simulink model "eVTOL_System"  (R2024b)
settings: Solver=FixedStepAuto  StartTime=0.0  StopTime=inf  RelTol=1e-3
undefined symbols (not defined in the file): airspeed, Battery, BCE12, BCE_Set_init, BMS_Controller_State, C, Cell10_P, Cell11_P, Cell12_P, Cell13_P, Cell14_P, Cell15_P, Cell16_P, Cell17_P, Cell18_P, Cell19_P, Cell1_N, Cell1_P, Cell20_P, Cell21_P, Cell22_P, Cell23_P, Cell24_P, Cell2_P, Cell3_P, Cell4_P, Cell5_P, Cell6_P, Cell7_P, Cell8_P, Cell9_P, Charging_State, CityMission, control, controlParams, ControlSampleTime, CriticalTiltAngle, currentFactor, CV_Gain, ddx, ddy, ddz, Device_01, Device_02, DiscIntNeverNeededParam, dx, dy, dz, Earth, env, F, F28379D_ADC_MaxCount, F28379D_ADC_Vmax, FixedWingMission, flightState, Foc_Ki_IxTcpu, Foc_Ki_S, Foc_Kp_I, Foc_Kp_S, fractalcoef ... (+68)
libraries: fl_lib x1115, nesl_utility x617, slrealtimeethercatlib x217, simulink x130, canmsglib x101, speedgoatlib_IO611_obsolete x91, slpidlib x49, mcbcontrolslib x44, slrealtimeutilitieslib x35, speedgoatlib_hdlCoder_IO3xx x31, dspstat3 x24, mcbpositiondecoderlib x12
(part 17 of 31)

== system eVTOL_System/Battery System/BMS/HIL/Controller_100Cells/PLANT-Rx/Messages ==
  ID_0x201 : Inport
  ID_0x202 : Inport  Port=2
  ID_0x501 : Inport  Port=3
  ID_0x502 : Inport  Port=4
  ID_0x203 : Inport  Port=5
  ID_0x204 : Inport  Port=6
  Balancing : simulink/Sources/Enumerated Constant  OutDataTypeStr=Enum: BMS_Controller_State  Value=BMS_Controller_State.BMS_Idle  SampleTime=-1
  Balancing1 : simulink/Sources/Enumerated Constant  OutDataTypeStr=Enum: Charging_State  Value=Charging_State.Init  SampleTime=-1
  Bus Creator : BusCreator  Inputs=5  OutDataTypeStr=Bus: Faults
  CAN Unpack : canmsglib/CAN Unpack  MsgList=(none)  MsgName=CAN Msg  MsgIDType=Standard (11-bit identifier)  MsgIdentifier=0x201  MsgLength=8  SignalInfo={ 'DischargeCurrentLimit_CAN', '0', '32', 'LE', 'single', 'Standard', '0', '1', '0', '-inf', '+inf'; 'ChargeCurrentLimit_CAN', '32', '32', 'LE', 'single', 'Standard', '0', '1', '0', '-Inf', 'Inf' }  IDPort=off  TimestampPort=on  ErrorPort=off  RemotePort=off  LengthPort=off  StatusPort=on  ApplyMinMax=off
      settings: LibrarySourceBlock=embeddedtargetslib/Host Communication/CAN Unpack
  CAN Unpack1 : canmsglib/CAN Unpack  MsgList=(none)  MsgName=CAN Msg  MsgIDType=Standard (11-bit identifier)  MsgIdentifier=0x202  MsgLength=4  SignalInfo={ 'ChargeCurrentReq', '0', '32', 'LE', 'single', 'Standard', '0', '1', '0', '-inf', '+inf' }  IDPort=off  TimestampPort=on  ErrorPort=off  RemotePort=off  LengthPort=off  StatusPort=on  ApplyMinMax=off
      settings: LibrarySourceBlock=embeddedtargetslib/Host Communication/CAN Unpack
  CAN Unpack2 : canmsglib/CAN Unpack  MsgList=(none)  MsgName=CAN Msg  MsgIDType=Standard (11-bit identifier)  MsgIdentifier=0x501  MsgLength=8  SignalInfo={ 'SOC_UKF', '0', '32', 'LE', 'single', 'Standard', '0', '1', '0', '-inf', '+inf'; 'SOC_EKF', '32', '32', 'LE', 'single', 'Standard', '0', '1', '0', '-Inf', 'Inf' }  IDPort=off  TimestampPort=on  ErrorPort=off  RemotePort=off  LengthPort=off  StatusPort=on  ApplyMinMax=off
      settings: LibrarySourceBlock=embeddedtargetslib/Host Communication/CAN Unpack
  CAN Unpack3 : canmsglib/CAN Unpack  MsgList=(none)  MsgName=CAN Msg  MsgIDType=Standard (11-bit identifier)  MsgIdentifier=0x502  MsgLength=7  SignalInfo={ 'SOC_CC', '0', '32', 'LE', 'single', 'Standard', '0', '1', '0', '-inf', '+inf'; 'Faults', '32', '8', 'LE', 'unsigned', 'Standard', '0', '1', '0', '-Inf', 'Inf'; 'BMS_State', '40', '8', 'LE', 'unsigned', 'Standard', '0', '1', '0', '-Inf', 'Inf'; 'Charging_State', '48', '8', 'LE', 'signed', 'Standard', '0', '1', '0', '-Inf', 'Inf' }  IDPort=off  TimestampPort=on  ErrorPort=off  RemotePort=off  LengthPort=off  StatusPort=on  ApplyMinMax=off
      settings: LibrarySourceBlock=embeddedtargetslib/Host Communication/CAN Unpack
  CAN Unpack4 : canmsglib/CAN Unpack  MsgList=(none)  MsgName=CAN Msg  MsgIDType=Standard (11-bit identifier)  MsgIdentifier=0x203  MsgLength=8  SignalInfo={ 'Bal_Cmd1', '0', '32', 'LE', 'single', 'Standard', '0', '1', '0', '-inf', '+inf'; 'Bal_Cmd2', '32', '32', 'LE', 'single', 'Standard', '0', '1', '0', '-Inf', 'Inf' }  IDPort=off  TimestampPort=on  ErrorPort=off  RemotePort=off  LengthPort=off  StatusPort=on  ApplyMinMax=off
      settings: LibrarySourceBlock=embeddedtargetslib/Host Communication/CAN Unpack
  CAN Unpack5 : canmsglib/CAN Unpack  MsgList=(none)  MsgName=CAN Msg  MsgIDType=Standard (11-bit identifier)  MsgIdentifier=0x204  MsgLength=4  SignalInfo={ 'Bal_Cmd3', '0', '32', 'LE', 'single', 'Standard', '0', '1', '0', '-inf', '+inf' }  IDPort=off  TimestampPort=on  ErrorPort=off  RemotePort=off  LengthPort=off  StatusPort=on  ApplyMinMax=off
      settings: LibrarySourceBlock=embeddedtargetslib/Host Communication/CAN Unpack
  Charging : simulink/Sources/Enumerated Constant  OutDataTypeStr=Enum: BMS_Controller_State  Value=BMS_Controller_State.BMS_Driving  SampleTime=-1
  Charging1 : simulink/Sources/Enumerated Constant  OutDataTypeStr=Enum: Charging_State  Value=Charging_State.CC  SampleTime=-1
  Driving : simulink/Sources/Enumerated Constant  OutDataTypeStr=Enum: BMS_Controller_State  Value=BMS_Controller_State.BMS_Charging  SampleTime=-1
  Driving1 : simulink/Sources/Enumerated Constant  OutDataTypeStr=Enum: BMS_Controller_State  Value=BMS_Controller_State.BMS_Fault  SampleTime=-1
  Driving2 : simulink/Sources/Enumerated Constant  OutDataTypeStr=Enum: Charging_State  Value=Charging_State.CV  SampleTime=-1
  Faults_unpacking : slrealtimeutilitieslib/Bit Unpacking  SignExtend=on  MaskBitPatterns={[7:7] [6:6] [5:5] [4:4] [3:3] [2:2] [1:1] [0:0]}  MaskPackDataType=uint8  MaskPackDataSize=[1]  MaskUnpackDataTypes={'boolean', 'boolean', 'boolean', 'boolean', 'boolean', 'boolean', 'boolean', 'boolean'}  MaskUnpackDataSizes={[1] [1] [1] [1] [1] [1] [1] [1]}
  Gain : Gain  Gain=100
  Gain1 : Gain  Gain=100
  Gain2 : Gain  Gain=100
  Multiport Switch1 : MultiPortSwitch  DataPortOrder=Zero-based contiguous  zeroidx=on  SaturateOnIntegerOverflow=off  InputSameDT=off
  Multiport Switch2 : MultiPortSwitch  DataPortOrder=Zero-based contiguous  Inputs=4  zeroidx=on  SaturateOnIntegerOverflow=off  InputSameDT=off
  Mux1 : Mux  Inputs=3
  Subsystem : Subsystem
  Terminator{,1..10,13..16} (15 alike) : Terminator
  Discharge_Current_Limit : Outport
  Charge_Current_Limit : Outport  Port=2
  Charge_Current_Req : Outport  Port=3
  SOC : Outport  Port=4
  BMS_Faults : Outport  Port=5
  BMS_State : Outport  Port=6
  Charging_State : Outport  Port=7
  Bal_Cmd_76Cells : Outport  Port=8
  wires:
  CAN Unpack1/2 -> Terminator2/1
  CAN Unpack/1 -> Discharge_Current_Limit/1  "Discharge_Current_Limit"
  CAN Unpack1/1 -> Charge_Current_Req/1  "Charge_Current_Req"
  CAN Unpack1/3 -> Terminator5/1
  CAN Unpack/2 -> Charge_Current_Limit/1  "Charge_Current_Limit"
  CAN Unpack/4 -> Terminator7/1
  CAN Unpack/3 -> Terminator4/1
  ID_0x201/1 -> CAN Unpack/1
  ID_0x202/1 -> CAN Unpack1/1
  CAN Unpack2/2 -> Gain1/1
  Bus Creator/1 -> BMS_Faults/1
  Faults_unpacking/5 -> Bus Creator/5  "UnderVolt"
  CAN Unpack3/5 -> Terminator10/1
  CAN Unpack3/3 -> Multiport Switch2/1
  CAN Unpack3/2 -> Faults_unpacking/1
  Faults_unpacking/4 -> Bus Creator/4  "OverVolt"
  Faults_unpacking/3 -> Bus Creator/3  "LowTemp"
  CAN Unpack2/1 -> Gain/1
  Faults_unpacking/1 -> Bus Creator/1  "OverCurrent"
  ID_0x501/1 -> CAN Unpack2/1
  Faults_unpacking/2 -> Bus Creator/2  "HighTemp"
  CAN Unpack2/3 -> Terminator/1  "Time_0x501"
  ID_0x502/1 -> CAN Unpack3/1
  Gain/1 -> Mux1/1  "SOC_UKF"
  Gain1/1 -> Mux1/2  "SOC_EKF"
  CAN Unpack3/1 -> Gain2/1
  CAN Unpack2/4 -> Terminator1/1  "Status_0x501"
  Faults_unpacking/6 -> Terminator13/1
  Faults_unpacking/7 -> Terminator14/1
  Faults_unpacking/8 -> Terminator15/1
  CAN Unpack3/6 -> Terminator16/1
  Gain2/1 -> Mux1/3  "SOC_CC"
  Mux1/1 -> SOC/1  "SOC"
  Charging/1 -> Multiport Switch2/3
  Balancing/1 -> Multiport Switch2/2
  Driving/1 -> Multiport Switch2/4
  Driving1/1 -> Multiport Switch2/5
  Charging1/1 -> Multiport Switch1/3
  Driving2/1 -> Multiport Switch1/4
  Balancing1/1 -> Multiport Switch1/2
  CAN Unpack3/4 -> Multiport Switch1/1
  Multiport Switch1/1 -> Charging_State/1
  Multiport Switch2/1 -> BMS_State/1
  ID_0x203/1 -> CAN Unpack4/1
  ID_0x204/1 -> CAN Unpack5/1
  CAN Unpack5/3 -> Terminator9/1
  CAN Unpack5/2 -> Terminator8/1
  CAN Unpack4/3 -> Terminator3/1
  CAN Unpack4/4 -> Terminator6/1
  CAN Unpack4/1 -> Subsystem/1(In1)
  CAN Unpack5/1 -> Subsystem/3(3)
  CAN Unpack4/2 -> Subsystem/2(In2)
  Subsystem/1(Bal_Cmd_76Cells) -> Bal_Cmd_76Cells/1

== system eVTOL_System/Battery System/BMS/HIL/Controller_100Cells/PLANT-Tx/24-Cell ==
  to_Controller : Inport
  to_Controller_SRE : Inport  Port=2
  100 cells Temperature : Subsystem
  76 cells Voltage : Subsystem
  Bus Selector : BusSelector  OutputSignals=Pack_Current,Cell_Temperatures,Pack_Voltage2
  CAN Pack4 : canmsglib/CAN Pack  MsgList=(none)  MsgName=CAN Msg  MsgIDType=Standard (11-bit identifier)  MsgIdentifier=0x401  CANIDInput=off  MsgLength=5  Remote=off  ApplyMinMax=off  BusOutput=off  SignalInfo={ 'Pack_Current', '0', '32', 'LE', 'single', 'Standard', '0', '1', '0', '-Inf', 'Inf'; 'SRE', '32', '8', 'LE', 'unsigned', 'Standard', '0', '1', '0', '-Inf', 'Inf' }
      settings: LibrarySourceBlock=embeddedtargetslib/Host Communication/CAN Pack  DataFormat=manually specified signals
  CAN Write : speedgoatlib_IO611_obsolete/CAN/CAN Write  id=1  sampleTime=-1  portSelection=2  messageType=CAN  BusInput=off  enaStatusPort=off  protl=IO611  ptIdx=1  isFDMod=1
      settings: SourceProductName=IO611
  Selector : Subsystem  Commented=on
  wires:
  to_Controller/1 -> Bus Selector/1
  Bus Selector/1 -> CAN Pack4/1  "<Pack_Current>"
  CAN Pack4/1 -> CAN Write/1
  to_Controller_SRE/1 -> CAN Pack4/2
  Bus Selector/2 -> 100 cells Temperature/1(In1)  "<Cell_Temperatures>"
  Bus Selector/3 -> 76 cells Voltage/1(In1)  "<Pack_Voltage2>"

== system eVTOL_System/Battery System/BMS/HIL/Controller_76Cells/BMS State Machine/Selector1 ==
  In1 : Inport
  Demux : Demux  Outputs=100
  Mux : Mux  Inputs=24
  Mux1 : Mux  Inputs=76
  Terminator : Terminator
  Out1 : Outport
  wires:
  In1/1 -> Demux/1
  Demux/1 -> Mux/1
  Demux/2 -> Mux/2
  Demux/3 -> Mux/3
  Demux/4 -> Mux/4
  Demux/5 -> Mux/5
  Demux/6 -> Mux/6
  Demux/7 -> Mux/7
  Demux/8 -> Mux/8
  Demux/9 -> Mux/9
  Demux/10 -> Mux/10
  Demux/11 -> Mux/11
  Demux/12 -> Mux/12
  Demux/13 -> Mux/13
  Demux/14 -> Mux/14
  Demux/15 -> Mux/15
  Demux/16 -> Mux/16
  Demux/17 -> Mux/17
  Demux/18 -> Mux/18
  Demux/19 -> Mux/19
  Demux/20 -> Mux/20
  Demux/21 -> Mux/21
  Demux/22 -> Mux/22
  Demux/23 -> Mux/23
  Demux/24 -> Mux/24
  Demux/25 -> Mux1/1
  Demux/26 -> Mux1/2
  Demux/27 -> Mux1/3
  Demux/28 -> Mux1/4
  Demux/29 -> Mux1/5
  Demux/30 -> Mux1/6
  Demux/31 -> Mux1/7
  Demux/32 -> Mux1/8
  Demux/33 -> Mux1/9
  Demux/34 -> Mux1/10
  Demux/35 -> Mux1/11
  Demux/36 -> Mux1/12
  Demux/37 -> Mux1/13
  Demux/38 -> Mux1/14
  Demux/39 -> Mux1/15
  Demux/40 -> Mux1/16
  Demux/41 -> Mux1/17
  Demux/42 -> Mux1/18
  Demux/43 -> Mux1/19
  Demux/44 -> Mux1/20
  Demux/45 -> Mux1/21
  Demux/46 -> Mux1/22
  Demux/47 -> Mux1/23
  Demux/48 -> Mux1/24
  Demux/49 -> Mux1/25
  Demux/50 -> Mux1/26
  Demux/51 -> Mux1/27
  Demux/52 -> Mux1/28
  Demux/53 -> Mux1/29
  Demux/54 -> Mux1/30
  Demux/55 -> Mux1/31
  Demux/56 -> Mux1/32
  Demux/57 -> Mux1/33
  Demux/58 -> Mux1/34
  Demux/59 -> Mux1/35
  Demux/60 -> Mux1/36
  Demux/61 -> Mux1/37
  Demux/62 -> Mux1/38
  Demux/63 -> Mux1/39
  Demux/64 -> Mux1/40
  Demux/65 -> Mux1/41
  Demux/66 -> Mux1/42
  Demux/67 -> Mux1/43
  Demux/68 -> Mux1/44
  Demux/69 -> Mux1/45
  Demux/70 -> Mux1/46
  Demux/71 -> Mux1/47
  Demux/72 -> Mux1/48
  Demux/73 -> Mux1/49
  Demux/74 -> Mux1/50
  Demux/75 -> Mux1/51
  Demux/76 -> Mux1/52
  Demux/77 -> Mux1/53
  Demux/78 -> Mux1/54
  Demux/79 -> Mux1/55
  Demux/80 -> Mux1/56
  Demux/81 -> Mux1/57
  Demux/82 -> Mux1/58
  Demux/83 -> Mux1/59
  Demux/84 -> Mux1/60
  Demux/85 -> Mux1/61
  Demux/86 -> Mux1/62
  Demux/87 -> Mux1/63
  Demux/88 -> Mux1/64
  Demux/89 -> Mux1/65
  Demux/90 -> Mux1/66
  Demux/91 -> Mux1/67
  Demux/92 -> Mux1/68
  Demux/93 -> Mux1/69
  Demux/94 -> Mux1/70
  Demux/95 -> Mux1/71
  Demux/96 -> Mux1/72
  Demux/97 -> Mux1/73
  Demux/98 -> Mux1/74
  Demux/99 -> Mux1/75
  Demux/100 -> Mux1/76
  Mux1/1 -> Out1/1
  Mux/1 -> Terminator/1

== system eVTOL_System/Battery System/BMS/HIL/Controller_76Cells/BMS State Machine/Selector3 ==
  In1 : Inport
  Demux : Demux  Outputs=100
  Mux : Mux  Inputs=24
  Mux1 : Mux  Inputs=76
  Terminator : Terminator
  Out1 : Outport
  wires:
  In1/1 -> Demux/1
  Demux/1 -> Mux/1
  Demux/2 -> Mux/2
  Demux/3 -> Mux/3
  Demux/4 -> Mux/4
  Demux/5 -> Mux/5
  Demux/6 -> Mux/6
  Demux/7 -> Mux/7
  Demux/8 -> Mux/8
  Demux/9 -> Mux/9
  Demux/10 -> Mux/10
  Demux/11 -> Mux/11
  Demux/12 -> Mux/12
  Demux/13 -> Mux/13
  Demux/14 -> Mux/14
  Demux/15 -> Mux/15
  Demux/16 -> Mux/16
  Demux/17 -> Mux/17
  Demux/18 -> Mux/18
  Demux/19 -> Mux/19
  Demux/20 -> Mux/20
  Demux/21 -> Mux/21
  Demux/22 -> Mux/22
  Demux/23 -> Mux/23
  Demux/24 -> Mux/24
  Demux/25 -> Mux1/1
  Demux/26 -> Mux1/2
  Demux/27 -> Mux1/3
  Demux/28 -> Mux1/4
  Demux/29 -> Mux1/5
  Demux/30 -> Mux1/6
  Demux/31 -> Mux1/7
  Demux/32 -> Mux1/8
  Demux/33 -> Mux1/9
  Demux/34 -> Mux1/10
  Demux/35 -> Mux1/11
  Demux/36 -> Mux1/12
  Demux/37 -> Mux1/13
  Demux/38 -> Mux1/14
  Demux/39 -> Mux1/15
  Demux/40 -> Mux1/16
  Demux/41 -> Mux1/17
  Demux/42 -> Mux1/18
  Demux/43 -> Mux1/19
  Demux/44 -> Mux1/20
  Demux/45 -> Mux1/21
  Demux/46 -> Mux1/22
  Demux/47 -> Mux1/23
  Demux/48 -> Mux1/24
  Demux/49 -> Mux1/25
  Demux/50 -> Mux1/26
  Demux/51 -> Mux1/27
  Demux/52 -> Mux1/28
  Demux/53 -> Mux1/29
  Demux/54 -> Mux1/30
  Demux/55 -> Mux1/31
  Demux/56 -> Mux1/32
  Demux/57 -> Mux1/33
  Demux/58 -> Mux1/34
  Demux/59 -> Mux1/35
  Demux/60 -> Mux1/36
  Demux/61 -> Mux1/37
  Demux/62 -> Mux1/38
  Demux/63 -> Mux1/39
  Demux/64 -> Mux1/40
  Demux/65 -> Mux1/41
  Demux/66 -> Mux1/42
  Demux/67 -> Mux1/43
  Demux/68 -> Mux1/44
  Demux/69 -> Mux1/45
  Demux/70 -> Mux1/46
  Demux/71 -> Mux1/47
  Demux/72 -> Mux1/48
  Demux/73 -> Mux1/49
  Demux/74 -> Mux1/50
  Demux/75 -> Mux1/51
  Demux/76 -> Mux1/52
  Demux/77 -> Mux1/53
  Demux/78 -> Mux1/54
  Demux/79 -> Mux1/55
  Demux/80 -> Mux1/56
  Demux/81 -> Mux1/57
  Demux/82 -> Mux1/58
  Demux/83 -> Mux1/59
  Demux/84 -> Mux1/60
  Demux/85 -> Mux1/61
  Demux/86 -> Mux1/62
  Demux/87 -> Mux1/63
  Demux/88 -> Mux1/64
  Demux/89 -> Mux1/65
  Demux/90 -> Mux1/66
  Demux/91 -> Mux1/67
  Demux/92 -> Mux1/68
  Demux/93 -> Mux1/69
  Demux/94 -> Mux1/70
  Demux/95 -> Mux1/71
  Demux/96 -> Mux1/72
  Demux/97 -> Mux1/73
  Demux/98 -> Mux1/74
  Demux/99 -> Mux1/75
  Demux/100 -> Mux1/76
  Mux1/1 -> Out1/1
  Mux/1 -> Terminator/1

== system eVTOL_System/Battery System/BMS/HIL/Controller_76Cells/Balancing Logic/Selector1 ==
  In1 : Inport
  Demux : Demux  Outputs=100
  Mux : Mux  Inputs=24
  Mux1 : Mux  Inputs=76
  Terminator : Terminator
  Out1 : Outport
  wires:
  In1/1 -> Demux/1
  Demux/1 -> Mux/1
  Demux/2 -> Mux/2
  Demux/3 -> Mux/3
  Demux/4 -> Mux/4
  Demux/5 -> Mux/5
  Demux/6 -> Mux/6
  Demux/7 -> Mux/7
  Demux/8 -> Mux/8
  Demux/9 -> Mux/9
  Demux/10 -> Mux/10
  Demux/11 -> Mux/11
  Demux/12 -> Mux/12
  Demux/13 -> Mux/13
  Demux/14 -> Mux/14
  Demux/15 -> Mux/15
  Demux/16 -> Mux/16
  Demux/17 -> Mux/17
  Demux/18 -> Mux/18
  Demux/19 -> Mux/19
  Demux/20 -> Mux/20
  Demux/21 -> Mux/21
  Demux/22 -> Mux/22
  Demux/23 -> Mux/23
  Demux/24 -> Mux/24
  Demux/25 -> Mux1/1
  Demux/26 -> Mux1/2
  Demux/27 -> Mux1/3
  Demux/28 -> Mux1/4
  Demux/29 -> Mux1/5
  Demux/30 -> Mux1/6
  Demux/31 -> Mux1/7
  Demux/32 -> Mux1/8
  Demux/33 -> Mux1/9
  Demux/34 -> Mux1/10
  Demux/35 -> Mux1/11
  Demux/36 -> Mux1/12
  Demux/37 -> Mux1/13
  Demux/38 -> Mux1/14
  Demux/39 -> Mux1/15
  Demux/40 -> Mux1/16
  Demux/41 -> Mux1/17
  Demux/42 -> Mux1/18
  Demux/43 -> Mux1/19
  Demux/44 -> Mux1/20
  Demux/45 -> Mux1/21
  Demux/46 -> Mux1/22
  Demux/47 -> Mux1/23
  Demux/48 -> Mux1/24
  Demux/49 -> Mux1/25
  Demux/50 -> Mux1/26
  Demux/51 -> Mux1/27
  Demux/52 -> Mux1/28
  Demux/53 -> Mux1/29
  Demux/54 -> Mux1/30
  Demux/55 -> Mux1/31
  Demux/56 -> Mux1/32
  Demux/57 -> Mux1/33
  Demux/58 -> Mux1/34
  Demux/59 -> Mux1/35
  Demux/60 -> Mux1/36
  Demux/61 -> Mux1/37
  Demux/62 -> Mux1/38
  Demux/63 -> Mux1/39
  Demux/64 -> Mux1/40
  Demux/65 -> Mux1/41
  Demux/66 -> Mux1/42
  Demux/67 -> Mux1/43
  Demux/68 -> Mux1/44
  Demux/69 -> Mux1/45
  Demux/70 -> Mux1/46
  Demux/71 -> Mux1/47
  Demux/72 -> Mux1/48
  Demux/73 -> Mux1/49
  Demux/74 -> Mux1/50
  Demux/75 -> Mux1/51
  Demux/76 -> Mux1/52
  Demux/77 -> Mux1/53
  Demux/78 -> Mux1/54
  Demux/79 -> Mux1/55
  Demux/80 -> Mux1/56
  Demux/81 -> Mux1/57
  Demux/82 -> Mux1/58
  Demux/83 -> Mux1/59
  Demux/84 -> Mux1/60
  Demux/85 -> Mux1/61
  Demux/86 -> Mux1/62
  Demux/87 -> Mux1/63
  Demux/88 -> Mux1/64
  Demux/89 -> Mux1/65
  Demux/90 -> Mux1/66
  Demux/91 -> Mux1/67
  Demux/92 -> Mux1/68
  Demux/93 -> Mux1/69
  Demux/94 -> Mux1/70
  Demux/95 -> Mux1/71
  Demux/96 -> Mux1/72
  Demux/97 -> Mux1/73
  Demux/98 -> Mux1/74
  Demux/99 -> Mux1/75
  Demux/100 -> Mux1/76
  Mux1/1 -> Out1/1
  Mux/1 -> Terminator/1

== system eVTOL_System/Battery System/BMS/HIL/Controller_76Cells/Current Calculations/Charge_Current_Limit_Calc ==
  MaxCellVolt : Inport
  MinCellTemp : Inport  Port=2
  MaxCellTemp : Inport  Port=3
  Divide1 : Product  Inputs=*/
  HighTempChrgCurrentLim : Lookup_n-D  NumberOfTableDimensions=1  BreakpointsForDimension1=273.15+[-30:1:70]  Table=50*(1-tanh(273.15+[-30:1:70]-273.15-50))/2  InternalRulePriority=Speed  RndMeth=Simplest
  InternalCellResistance : Constant  Value=single(max(max(Battery(1).R0_LUT)))  OutDataTypeStr=single  SampleTime=-1
  LowTempChrgCurrentLim : Lookup_n-D  NumberOfTableDimensions=1  BreakpointsForDimension1=273.15+[-30:1:70]  Table=50*(1+tanh(273.15+[-30:1:70]-(273.15)))/2  InternalRulePriority=Speed  RndMeth=Simplest
  MinMax2 : MinMax  Inputs=3
  OverVoltageLimit : Constant  Value=OverCellVoltageLimit  OutDataTypeStr=single  SampleTime=-1
  Subtract1 : Sum  Inputs=+-
  Charge_Current_Limit : Outport  VectorParamsAs1DForOutWhenUnconnected=off
  wires:
  OverVoltageLimit/1 -> Subtract1/1
  MinMax2/1 -> Charge_Current_Limit/1  "ChargeCurrentLimit"
  MaxCellVolt/1 -> Subtract1/2
  Subtract1/1 -> Divide1/1
  Divide1/1 -> MinMax2/1
  InternalCellResistance/1 -> Divide1/2
  MinCellTemp/1 -> LowTempChrgCurrentLim/1
  MaxCellTemp/1 -> HighTempChrgCurrentLim/1
  HighTempChrgCurrentLim/1 -> MinMax2/3
  LowTempChrgCurrentLim/1 -> MinMax2/2

== system eVTOL_System/Battery System/BMS/HIL/Controller_76Cells/Current Calculations/Discharge_Current_Limit_Calc ==
  MinCellVolt : Inport
  MinCellTemp : Inport  Port=2
  MaxCellTemp : Inport  Port=3
  Divide : Product  Inputs=*/
  Gain : Gain  Gain=-1
  HighTempDchrgCurrentLim : Lookup_n-D  NumberOfTableDimensions=1  BreakpointsForDimension1=273.15+[-30:1:70]  Table=100*(1-tanh(273.15+[-30:1:70]-273.15-50))/2  InternalRulePriority=Speed  RndMeth=Simplest
  InternalCellResistance : Constant  Value=single(max(max(Battery(1).R0_LUT)))  OutDataTypeStr=single  SampleTime=-1
  LowTempDchrgCurrentLim : Lookup_n-D  NumberOfTableDimensions=1  BreakpointsForDimension1=273.15+[-30:1:70]  Table=100*(1+tanh(273.15+[-30:1:70]-(273.15)))/2  InternalRulePriority=Speed  RndMeth=Simplest
  MinMax2 : MinMax  Inputs=3
  Subtract : Sum  Inputs=+-
  UnderVoltageLimit : Constant  Value=UnderCellVoltageLimit  OutDataTypeStr=single  SampleTime=-1
  Discharge_Current_Limit : Outport  VectorParamsAs1DForOutWhenUnconnected=off
  wires:
  MinMax2/1 -> Gain/1  "DischargeCurrentLimit"
  Divide/1 -> MinMax2/1
  MinCellVolt/1 -> Subtract/1
  InternalCellResistance/1 -> Divide/2
  Subtract/1 -> Divide/1
  UnderVoltageLimit/1 -> Subtract/2
  Gain/1 -> Discharge_Current_Limit/1
  MaxCellTemp/1 -> HighTempDchrgCurrentLim/1
  MinCellTemp/1 -> LowTempDchrgCurrentLim/1
  HighTempDchrgCurrentLim/1 -> MinMax2/3
  LowTempDchrgCurrentLim/1 -> MinMax2/2

== system eVTOL_System/Battery System/BMS/HIL/Controller_76Cells/Current Calculations/Selector1 ==
  In1 : Inport
  Demux : Demux  Outputs=100
  Mux : Mux  Inputs=24
  Mux1 : Mux  Inputs=76
  Terminator : Terminator
  Out1 : Outport
  wires:
  In1/1 -> Demux/1
  Demux/1 -> Mux/1
  Demux/2 -> Mux/2
  Demux/3 -> Mux/3
  Demux/4 -> Mux/4
  Demux/5 -> Mux/5
  Demux/6 -> Mux/6
  Demux/7 -> Mux/7
  Demux/8 -> Mux/8
  Demux/9 -> Mux/9
  Demux/10 -> Mux/10
  Demux/11 -> Mux/11
  Demux/12 -> Mux/12
  Demux/13 -> Mux/13
  Demux/14 -> Mux/14
  Demux/15 -> Mux/15
  Demux/16 -> Mux/16
  Demux/17 -> Mux/17
  Demux/18 -> Mux/18
  Demux/19 -> Mux/19
  Demux/20 -> Mux/20
  Demux/21 -> Mux/21
  Demux/22 -> Mux/22
  Demux/23 -> Mux/23
  Demux/24 -> Mux/24
  Demux/25 -> Mux1/1
  Demux/26 -> Mux1/2
  Demux/27 -> Mux1/3
  Demux/28 -> Mux1/4
  Demux/29 -> Mux1/5
  Demux/30 -> Mux1/6
  Demux/31 -> Mux1/7
  Demux/32 -> Mux1/8
  Demux/33 -> Mux1/9
  Demux/34 -> Mux1/10
  Demux/35 -> Mux1/11
  Demux/36 -> Mux1/12
  Demux/37 -> Mux1/13
  Demux/38 -> Mux1/14
  Demux/39 -> Mux1/15
  Demux/40 -> Mux1/16
  Demux/41 -> Mux1/17
  Demux/42 -> Mux1/18
  Demux/43 -> Mux1/19
  Demux/44 -> Mux1/20
  Demux/45 -> Mux1/21
  Demux/46 -> Mux1/22
  Demux/47 -> Mux1/23
  Demux/48 -> Mux1/24
  Demux/49 -> Mux1/25
  Demux/50 -> Mux1/26
  Demux/51 -> Mux1/27
  Demux/52 -> Mux1/28
  Demux/53 -> Mux1/29
  Demux/54 -> Mux1/30
  Demux/55 -> Mux1/31
  Demux/56 -> Mux1/32
  Demux/57 -> Mux1/33
  Demux/58 -> Mux1/34
  Demux/59 -> Mux1/35
  Demux/60 -> Mux1/36
  Demux/61 -> Mux1/37
  Demux/62 -> Mux1/38
  Demux/63 -> Mux1/39
  Demux/64 -> Mux1/40
  Demux/65 -> Mux1/41
  Demux/66 -> Mux1/42
  Demux/67 -> Mux1/43
  Demux/68 -> Mux1/44
  Demux/69 -> Mux1/45
  Demux/70 -> Mux1/46
  Demux/71 -> Mux1/47
  Demux/72 -> Mux1/48
  Demux/73 -> Mux1/49
  Demux/74 -> Mux1/50
  Demux/75 -> Mux1/51
  Demux/76 -> Mux1/52
  Demux/77 -> Mux1/53
  Demux/78 -> Mux1/54
  Demux/79 -> Mux1/55
  Demux/80 -> Mux1/56
  Demux/81 -> Mux1/57
  Demux/82 -> Mux1/58
  Demux/83 -> Mux1/59
  Demux/84 -> Mux1/60
  Demux/85 -> Mux1/61
  Demux/86 -> Mux1/62
  Demux/87 -> Mux1/63
  Demux/88 -> Mux1/64
  Demux/89 -> Mux1/65
  Demux/90 -> Mux1/66
  Demux/91 -> Mux1/67
  Demux/92 -> Mux1/68
  Demux/93 -> Mux1/69
  Demux/94 -> Mux1/70
  Demux/95 -> Mux1/71
  Demux/96 -> Mux1/72
  Demux/97 -> Mux1/73
  Demux/98 -> Mux1/74
  Demux/99 -> Mux1/75
  Demux/100 -> Mux1/76
  Mux1/1 -> Out1/1
  Mux/1 -> Terminator/1

== system eVTOL_System/Battery System/BMS/HIL/Controller_76Cells/Current Calculations/Selector3 ==
  In1 : Inport
  Demux : Demux  Outputs=100
  Mux : Mux  Inputs=24
  Mux1 : Mux  Inputs=76
  Terminator : Terminator
  Out1 : Outport
  wires:
  In1/1 -> Demux/1
  Demux/1 -> Mux/1
  Demux/2 -> Mux/2
  Demux/3 -> Mux/3
  Demux/4 -> Mux/4
  Demux/5 -> Mux/5
  Demux/6 -> Mux/6
  Demux/7 -> Mux/7
  Demux/8 -> Mux/8
  Demux/9 -> Mux/9
  Demux/10 -> Mux/10
  Demux/11 -> Mux/11
  Demux/12 -> Mux/12
  Demux/13 -> Mux/13
  Demux/14 -> Mux/14
  Demux/15 -> Mux/15
  Demux/16 -> Mux/16
  Demux/17 -> Mux/17
  Demux/18 -> Mux/18
  Demux/19 -> Mux/19
  Demux/20 -> Mux/20
  Demux/21 -> Mux/21
  Demux/22 -> Mux/22
  Demux/23 -> Mux/23
  Demux/24 -> Mux/24
  Demux/25 -> Mux1/1
  Demux/26 -> Mux1/2
  Demux/27 -> Mux1/3
  Demux/28 -> Mux1/4
  Demux/29 -> Mux1/5
  Demux/30 -> Mux1/6
  Demux/31 -> Mux1/7
  Demux/32 -> Mux1/8
  Demux/33 -> Mux1/9
  Demux/34 -> Mux1/10
  Demux/35 -> Mux1/11
  Demux/36 -> Mux1/12
  Demux/37 -> Mux1/13
  Demux/38 -> Mux1/14
  Demux/39 -> Mux1/15
  Demux/40 -> Mux1/16
  Demux/41 -> Mux1/17
  Demux/42 -> Mux1/18
  Demux/43 -> Mux1/19
  Demux/44 -> Mux1/20
  Demux/45 -> Mux1/21
  Demux/46 -> Mux1/22
  Demux/47 -> Mux1/23
  Demux/48 -> Mux1/24
  Demux/49 -> Mux1/25
  Demux/50 -> Mux1/26
  Demux/51 -> Mux1/27
  Demux/52 -> Mux1/28
  Demux/53 -> Mux1/29
  Demux/54 -> Mux1/30
  Demux/55 -> Mux1/31
  Demux/56 -> Mux1/32
  Demux/57 -> Mux1/33
  Demux/58 -> Mux1/34
  Demux/59 -> Mux1/35
  Demux/60 -> Mux1/36
  Demux/61 -> Mux1/37
  Demux/62 -> Mux1/38
  Demux/63 -> Mux1/39
  Demux/64 -> Mux1/40
  Demux/65 -> Mux1/41
  Demux/66 -> Mux1/42
  Demux/67 -> Mux1/43
  Demux/68 -> Mux1/44
  Demux/69 -> Mux1/45
  Demux/70 -> Mux1/46
  Demux/71 -> Mux1/47
  Demux/72 -> Mux1/48
  Demux/73 -> Mux1/49
  Demux/74 -> Mux1/50
  Demux/75 -> Mux1/51
  Demux/76 -> Mux1/52
  Demux/77 -> Mux1/53
  Demux/78 -> Mux1/54
  Demux/79 -> Mux1/55
  Demux/80 -> Mux1/56
  Demux/81 -> Mux1/57
  Demux/82 -> Mux1/58
  Demux/83 -> Mux1/59
  Demux/84 -> Mux1/60
  Demux/85 -> Mux1/61
  Demux/86 -> Mux1/62
  Demux/87 -> Mux1/63
  Demux/88 -> Mux1/64
  Demux/89 -> Mux1/65
  Demux/90 -> Mux1/66
  Demux/91 -> Mux1/67
  Demux/92 -> Mux1/68
  Demux/93 -> Mux1/69
  Demux/94 -> Mux1/70
  Demux/95 -> Mux1/71
  Demux/96 -> Mux1/72
  Demux/97 -> Mux1/73
  Demux/98 -> Mux1/74
  Demux/99 -> Mux1/75
  Demux/100 -> Mux1/76
  Mux1/1 -> Out1/1
  Mux/1 -> Terminator/1

== system eVTOL_System/Battery System/BMS/HIL/Controller_76Cells/SOC Calculation/Coulomb Counting ==
  Curr : Inport
  Temp : Inport  Port=2
  1-D Lookup Table : Lookup_n-D  NumberOfTableDimensions=1  BreakpointsForDimension1=single(Battery(1).Temperature_LUT)  Table=single(Battery(1).Capacity_LUT)  InternalRulePriority=Speed  RndMeth=Simplest
  Discrete-Time Integrator : DiscreteIntegrator  InitialCondition=single(SOCInit+0.05)  SampleTime=-1  LimitOutput=on  UpperSaturationLimit=1  LowerSaturationLimit=0  ICPrevOutput=DiscIntNeverNeededParam  ICPrevScaledInput=DiscIntNeverNeededParam
  Divide : Product  Inputs=*/
  Gain : Gain  Gain=single(1/3600)
  SOC : Outport  VectorParamsAs1DForOutWhenUnconnected=off
  wires:
  Discrete-Time Integrator/1 -> SOC/1
  Curr/1 -> Gain/1
  Gain/1 -> Divide/1
  Divide/1 -> Discrete-Time Integrator/1
  1-D Lookup Table/1 -> Divide/2  "Capacity"
  Temp/1 -> 1-D Lookup Table/1

== system eVTOL_System/Battery System/BMS/HIL/Controller_76Cells/SOC Calculation/Measurement Function ==
  Current : Inport
  Temperature (K) : Inport  Port=2
  batteryMeasurementFcn : TriggerPort  TriggerType=function-call  IsSimulinkFunction=on  FunctionName=batteryMeasurementFcn  VariantControl=Variant
  Add1 : Sum  Inputs=+--
  Em Table : Lookup_n-D  BreakpointsForDimension1=Battery.SOC_LUT  BreakpointsForDimension2=Battery.Temperature_LUT  BeginIndexSearchUsingPreviousIndexResult=on  Table=Battery.Em_LUT  ExtrapMethod=Clip  InternalRulePriority=Speed  RndMeth=Simplest
      settings: InputPortMap=u0,u1
  Get SOC : Selector  InputPortWidth=2  IndexOptions=Index vector (dialog)  Indices=[1]  OutputSizes=1
  Get U1 : Selector  InputPortWidth=2  IndexOptions=Index vector (dialog)  Indices=2  OutputSizes=1
  Product : Product
  R0 Table : Lookup_n-D  BreakpointsForDimension1=Battery.SOC_LUT  BreakpointsForDimension2=Battery.Temperature_LUT  BeginIndexSearchUsingPreviousIndexResult=on  Table=Battery.R0_LUT  ExtrapMethod=Clip  InternalRulePriority=Speed  RndMeth=Simplest
      settings: InputPortMap=u0,u1
  x : ArgIn  DisableCoverage=on  OutDataTypeStr=single  PortDimensions=2  ArgumentName=x
  y : ArgOut  DisableCoverage=on  OutDataTypeStr=single  ArgumentName=y
  wires:
  Get U1/1 -> Add1/3  "U1"
  Product/1 -> Add1/2
  Current/1 -> Product/2
  R0 Table/1 -> Product/1
  Temperature (K)/1 -> Em Table/2, R0 Table/2
  Add1/1 -> y/1
  Em Table/1 -> Add1/1
  Get SOC/1 -> Em Table/1, R0 Table/1  "SOC"
  x/1 -> Get SOC/1, Get U1/1

== system eVTOL_System/Battery System/BMS/HIL/Controller_76Cells/SOC Calculation/Selector ==
  In1 : Inport
  Demux : Demux  Outputs=100
  Mux : Mux  Inputs=24
  Mux1 : Mux  Inputs=76
  Terminator : Terminator
  Out1 : Outport
  wires:
  In1/1 -> Demux/1
  Demux/1 -> Mux/1
  Demux/2 -> Mux/2
  Demux/3 -> Mux/3
  Demux/4 -> Mux/4
  Demux/5 -> Mux/5
  Demux/6 -> Mux/6
  Demux/7 -> Mux/7
  Demux/8 -> Mux/8
  Demux/9 -> Mux/9
  Demux/10 -> Mux/10
  Demux/11 -> Mux/11
  Demux/12 -> Mux/12
  Demux/13 -> Mux/13
  Demux/14 -> Mux/14
  Demux/15 -> Mux/15
  Demux/16 -> Mux/16
  Demux/17 -> Mux/17
  Demux/18 -> Mux/18
  Demux/19 -> Mux/19
  Demux/20 -> Mux/20
  Demux/21 -> Mux/21
  Demux/22 -> Mux/22
  Demux/23 -> Mux/23
  Demux/24 -> Mux/24
  Demux/25 -> Mux1/1
  Demux/26 -> Mux1/2
  Demux/27 -> Mux1/3
  Demux/28 -> Mux1/4
  Demux/29 -> Mux1/5
  Demux/30 -> Mux1/6
  Demux/31 -> Mux1/7
  Demux/32 -> Mux1/8
  Demux/33 -> Mux1/9
  Demux/34 -> Mux1/10
  Demux/35 -> Mux1/11
  Demux/36 -> Mux1/12
  Demux/37 -> Mux1/13
  Demux/38 -> Mux1/14
  Demux/39 -> Mux1/15
  Demux/40 -> Mux1/16
  Demux/41 -> Mux1/17
  Demux/42 -> Mux1/18
  Demux/43 -> Mux1/19
  Demux/44 -> Mux1/20
  Demux/45 -> Mux1/21
  Demux/46 -> Mux1/22
  Demux/47 -> Mux1/23
  Demux/48 -> Mux1/24
  Demux/49 -> Mux1/25
  Demux/50 -> Mux1/26
  Demux/51 -> Mux1/27
  Demux/52 -> Mux1/28
  Demux/53 -> Mux1/29
  Demux/54 -> Mux1/30
  Demux/55 -> Mux1/31
  Demux/56 -> Mux1/32
  Demux/57 -> Mux1/33
  Demux/58 -> Mux1/34
  Demux/59 -> Mux1/35
  Demux/60 -> Mux1/36
  Demux/61 -> Mux1/37
  Demux/62 -> Mux1/38
  Demux/63 -> Mux1/39
  Demux/64 -> Mux1/40
  Demux/65 -> Mux1/41
  Demux/66 -> Mux1/42
  Demux/67 -> Mux1/43
  Demux/68 -> Mux1/44
  Demux/69 -> Mux1/45
  Demux/70 -> Mux1/46
  Demux/71 -> Mux1/47
  Demux/72 -> Mux1/48
  Demux/73 -> Mux1/49
  Demux/74 -> Mux1/50
  Demux/75 -> Mux1/51
  Demux/76 -> Mux1/52
  Demux/77 -> Mux1/53
  Demux/78 -> Mux1/54
  Demux/79 -> Mux1/55
  Demux/80 -> Mux1/56
  Demux/81 -> Mux1/57
  Demux/82 -> Mux1/58
  Demux/83 -> Mux1/59
  Demux/84 -> Mux1/60
  Demux/85 -> Mux1/61
  Demux/86 -> Mux1/62
  Demux/87 -> Mux1/63
  Demux/88 -> Mux1/64
  Demux/89 -> Mux1/65
  Demux/90 -> Mux1/66
  Demux/91 -> Mux1/67
  Demux/92 -> Mux1/68
  Demux/93 -> Mux1/69
  Demux/94 -> Mux1/70
  Demux/95 -> Mux1/71
  Demux/96 -> Mux1/72
  Demux/97 -> Mux1/73
  Demux/98 -> Mux1/74
  Demux/99 -> Mux1/75
  Demux/100 -> Mux1/76
  Mux1/1 -> Out1/1
  Mux/1 -> Terminator/1

== system eVTOL_System/Battery System/BMS/HIL/Controller_76Cells/SOC Calculation/Selector1 ==
  In1 : Inport
  Demux : Demux  Outputs=100
  Mux : Mux  Inputs=24
  Mux1 : Mux  Inputs=76
  Terminator : Terminator
  Out1 : Outport
  wires:
  In1/1 -> Demux/1
  Demux/1 -> Mux/1
  Demux/2 -> Mux/2
  Demux/3 -> Mux/3
  Demux/4 -> Mux/4
  Demux/5 -> Mux/5
  Demux/6 -> Mux/6
  Demux/7 -> Mux/7
  Demux/8 -> Mux/8
  Demux/9 -> Mux/9
  Demux/10 -> Mux/10
  Demux/11 -> Mux/11
  Demux/12 -> Mux/12
  Demux/13 -> Mux/13
  Demux/14 -> Mux/14
  Demux/15 -> Mux/15
  Demux/16 -> Mux/16
  Demux/17 -> Mux/17
  Demux/18 -> Mux/18
  Demux/19 -> Mux/19
  Demux/20 -> Mux/20
  Demux/21 -> Mux/21
  Demux/22 -> Mux/22
  Demux/23 -> Mux/23
  Demux/24 -> Mux/24
  Demux/25 -> Mux1/1
  Demux/26 -> Mux1/2
  Demux/27 -> Mux1/3
  Demux/28 -> Mux1/4
  Demux/29 -> Mux1/5
  Demux/30 -> Mux1/6
  Demux/31 -> Mux1/7
  Demux/32 -> Mux1/8
  Demux/33 -> Mux1/9
  Demux/34 -> Mux1/10
  Demux/35 -> Mux1/11
  Demux/36 -> Mux1/12
  Demux/37 -> Mux1/13
  Demux/38 -> Mux1/14
  Demux/39 -> Mux1/15
  Demux/40 -> Mux1/16
  Demux/41 -> Mux1/17
  Demux/42 -> Mux1/18
  Demux/43 -> Mux1/19
  Demux/44 -> Mux1/20
  Demux/45 -> Mux1/21
  Demux/46 -> Mux1/22
  Demux/47 -> Mux1/23
  Demux/48 -> Mux1/24
  Demux/49 -> Mux1/25
  Demux/50 -> Mux1/26
  Demux/51 -> Mux1/27
  Demux/52 -> Mux1/28
  Demux/53 -> Mux1/29
  Demux/54 -> Mux1/30
  Demux/55 -> Mux1/31
  Demux/56 -> Mux1/32
  Demux/57 -> Mux1/33
  Demux/58 -> Mux1/34
  Demux/59 -> Mux1/35
  Demux/60 -> Mux1/36
  Demux/61 -> Mux1/37
  Demux/62 -> Mux1/38
  Demux/63 -> Mux1/39
  Demux/64 -> Mux1/40
  Demux/65 -> Mux1/41
  Demux/66 -> Mux1/42
  Demux/67 -> Mux1/43
  Demux/68 -> Mux1/44
  Demux/69 -> Mux1/45
  Demux/70 -> Mux1/46
  Demux/71 -> Mux1/47
  Demux/72 -> Mux1/48
  Demux/73 -> Mux1/49
  Demux/74 -> Mux1/50
  Demux/75 -> Mux1/51
  Demux/76 -> Mux1/52
  Demux/77 -> Mux1/53
  Demux/78 -> Mux1/54
  Demux/79 -> Mux1/55
  Demux/80 -> Mux1/56
  Demux/81 -> Mux1/57
  Demux/82 -> Mux1/58
  Demux/83 -> Mux1/59
  Demux/84 -> Mux1/60
  Demux/85 -> Mux1/61
  Demux/86 -> Mux1/62
  Demux/87 -> Mux1/63
  Demux/88 -> Mux1/64
  Demux/89 -> Mux1/65
  Demux/90 -> Mux1/66
  Demux/91 -> Mux1/67
  Demux/92 -> Mux1/68
  Demux/93 -> Mux1/69
  Demux/94 -> Mux1/70
  Demux/95 -> Mux1/71
  Demux/96 -> Mux1/72
  Demux/97 -> Mux1/73
  Demux/98 -> Mux1/74
  Demux/99 -> Mux1/75
  Demux/100 -> Mux1/76
  Mux1/1 -> Out1/1
  Mux/1 -> Terminator/1

== system eVTOL_System/Battery System/BMS/HIL/Controller_76Cells/SOC Calculation/State Transition Function ==
  Current : Inport
  Temperature K : Inport  Port=2
  batteryStateFcn : TriggerPort  TriggerType=function-call  IsSimulinkFunction=on  FunctionName=batteryStateFcn  VariantControl=Variant
  Add : Sum
  Add1 : Sum  Inputs=-+
  C1 : Lookup_n-D  BreakpointsForDimension1=Battery.SOC_LUT  BreakpointsForDimension2=Battery.Temperature_LUT  BeginIndexSearchUsingPreviousIndexResult=on  Table=Battery.C1_LUT  ExtrapMethod=Clip  InternalRulePriority=Speed  RndMeth=Simplest
      settings: InputPortMap=u0,u1
  Constant : Constant  Value=single(ts_system)  OutDataTypeStr=single
  Divide : Product  Inputs=*/
  Divide1 : Product  Inputs=*/
  Divide2 : Product  Inputs=*/
  Gain : Gain  Gain=-3600
  Get SOC : Selector  InputPortWidth=2  IndexOptions=Index vector (dialog)  Indices=1  OutputSizes=1
  Get U1 : Selector  InputPortWidth=2  IndexOptions=Index vector (dialog)  Indices=2  OutputSizes=1
  Lookup Table : Lookup_n-D  NumberOfTableDimensions=1  BreakpointsForDimension1=Battery.Temperature_LUT  BeginIndexSearchUsingPreviousIndexResult=on  Table=Battery.Capacity_LUT  InternalRulePriority=Speed  RndMeth=Simplest
  Mux : Mux  Inputs=2
  Product : Product  OutDataTypeStr=single
  Product1 : Product
  R1 : Lookup_n-D  BreakpointsForDimension1=Battery.SOC_LUT  BreakpointsForDimension2=Battery.Temperature_LUT  BeginIndexSearchUsingPreviousIndexResult=on  Table=Battery.R1_LUT  ExtrapMethod=Clip  InternalRulePriority=Speed  RndMeth=Simplest
      settings: InputPortMap=u0,u1
  x : ArgIn  DisableCoverage=on  OutDataTypeStr=single  PortDimensions=2  ArgumentName=x
  xNext : ArgOut  DisableCoverage=on  OutDataTypeStr=single  PortDimensions=2  ArgumentName=xNext
  wires:
  Lookup Table/1 -> Gain/1  "Cq"
  Product/1 -> Add/2
  Constant/1 -> Product/2
  Current/1 -> Divide1/1, Divide/1  "Current"
  Get SOC/1 -> C1/1, R1/1
  Temperature K/1 -> Lookup Table/1, C1/2, R1/2
  Add/1 -> xNext/1
  x/1 -> Add/1, Get U1/1, Get SOC/1
  Gain/1 -> Divide/2
  Divide/1 -> Mux/1  "xdot_1"
  Get U1/1 -> Divide2/1  "U1"
  Product1/1 -> Divide2/2  "R1*C1"
  R1/1 -> Product1/1  "R1"
  C1/1 -> Product1/2, Divide1/2  "C1"
  Divide1/1 -> Add1/2  "Current/C1"
  Divide2/1 -> Add1/1
  Add1/1 -> Mux/2  "xdot_2"
  Mux/1 -> Product/1  "xdot"

== system eVTOL_System/Battery System/BMS/HIL/Controller_76Cells/SOC Calculation/UKF_EKF_1TC ==
  Cell_Voltage : Inport
  Enable : EnablePort
  EKF : sharedTrackingLibrary/Extended Kalman Filter  StateTransitionFcn=batteryStateFcn  HasStateTransitionJacobianFcn=off  HasAdditiveProcessNoise=Additive  ProcessNoise=1e-10*eye(2)  HasTimeVaryingProcessNoise=off  HasStateTransitionFcnExtraArgument=0  InitialState=[single(SOCInit+0.05); 0;]  InitialStateCovariance=[1e-5 1]  MeasurementFcn1=batteryMeasurementFcn  HasMeasurementJacobianFcn1=off  HasMeasurementEnablePort1=off  HasAdditiveMeasurementNoise1=Additive  MeasurementNoise1=1e-1  HasTimeVaryingMeasurementNoise1=off  HasMeasurementFcnExtraArgument1=0  HasMeasurementWrapping1=off  MeasurementFcn2=myMeasurementFcn  HasMeasurementJacobianFcn2=off  HasMeasurementEnablePort2=off  HasAdditiveMeasurementNoise2=Additive  MeasurementNoise2=1  HasTimeVaryingMeasurementNoise2=off  HasMeasurementFcnExtraArgument2=0  HasMeasurementWrapping2=off  MeasurementFcn3=myMeasurementFcn  HasMeasurementJacobianFcn3=off  HasMeasurementEnablePort3=off  HasAdditiveMeasurementNoise3=Additive  MeasurementNoise3=1  HasTimeVaryingMeasurementNoise3=off  HasMeasurementFcnExtraArgument3=0  HasMeasurementWrapping3=off  MeasurementFcn4=myMeasurementFcn  HasMeasurementJacobianFcn4=off  HasMeasurementEnablePort4=off  HasAdditiveMeasurementNoise4=Additive  MeasurementNoise4=1  HasTimeVaryingMeasurementNoise4=off  HasMeasurementFcnExtraArgument4=0  HasMeasurementWrapping4=off  MeasurementFcn5=myMeasurementFcn  HasMeasurementJacobianFcn5=off  HasMeasurementEnablePort5=off  HasAdditiveMeasurementNoise5=Additive  MeasurementNoise5=1  HasTimeVaryingMeasurementNoise5=off  HasMeasurementFcnExtraArgument5=0  HasMeasurementWrapping5=off  EnableMultirate=off  StateTransitionFcnSampleTime=1  MeasurementFcn1SampleTime=1  MeasurementFcn2SampleTime=1  MeasurementFcn3SampleTime=1  MeasurementFcn4SampleTime=1  MeasurementFcn5SampleTime=1  UseCurrentEstimator=on  OutputStateCovariance=off  DataType=single  SampleTime=ts_controller  NumberOfMeasurements=1
  SOC : Selector  InputPortWidth=2  IndexOptions=Index vector (dialog)  Indices=1  OutputSizes=1
  SOC1 : Selector  InputPortWidth=2  IndexOptions=Index vector (dialog)  Indices=1  OutputSizes=1
  UKF : sharedTrackingLibrary/Unscented Kalman Filter  StateTransitionFcn=batteryStateFcn  HasAdditiveProcessNoise=Additive  ProcessNoise=1e-10*eye(2)  HasTimeVaryingProcessNoise=off  HasStateTransitionFcnExtraArgument=0  InitialState=[single(SOCInit+0.05); 0;]  InitialStateCovariance=[1e-5 1]  Alpha=1  Beta=2  Kappa=1  MeasurementFcn1=batteryMeasurementFcn  HasMeasurementEnablePort1=off  HasAdditiveMeasurementNoise1=Additive  MeasurementNoise1=0.1  HasTimeVaryingMeasurementNoise1=off  HasMeasurementFcnExtraArgument1=0  HasMeasurementWrapping1=off  MeasurementFcn2=myMeasurementFcn  HasMeasurementEnablePort2=off  HasAdditiveMeasurementNoise2=Additive  MeasurementNoise2=1  HasTimeVaryingMeasurementNoise2=off  HasMeasurementFcnExtraArgument2=0  HasMeasurementWrapping2=off  MeasurementFcn3=myMeasurementFcn  HasMeasurementEnablePort3=off  HasAdditiveMeasurementNoise3=Additive  MeasurementNoise3=1  HasTimeVaryingMeasurementNoise3=off  HasMeasurementFcnExtraArgument3=0  HasMeasurementWrapping3=off  MeasurementFcn4=myMeasurementFcn  HasMeasurementEnablePort4=off  HasAdditiveMeasurementNoise4=Additive  MeasurementNoise4=1  HasTimeVaryingMeasurementNoise4=off  HasMeasurementFcnExtraArgument4=0  HasMeasurementWrapping4=off  MeasurementFcn5=myMeasurementFcn  HasMeasurementEnablePort5=off  HasAdditiveMeasurementNoise5=Additive  MeasurementNoise5=1  HasTimeVaryingMeasurementNoise5=off  HasMeasurementFcnExtraArgument5=0  HasMeasurementWrapping5=off  EnableMultirate=off  StateTransitionFcnSampleTime=-1  MeasurementFcn1SampleTime=-1  MeasurementFcn2SampleTime=-1  MeasurementFcn3SampleTime=-1  MeasurementFcn4SampleTime=-1  MeasurementFcn5SampleTime=-1  UseCurrentEstimator=on  OutputStateCovariance=off  DataType=single  SampleTime=ts_controller  NumberOfMeasurements=1
  SOC_UKF : Outport  VectorParamsAs1DForOutWhenUnconnected=off
  SOC_EKF : Outport  Port=2  VectorParamsAs1DForOutWhenUnconnected=off
  wires:
  UKF/1 -> SOC1/1
  Cell_Voltage/1 -> UKF/1, EKF/1
  SOC1/1 -> SOC_UKF/1  "SOC_UKF"
  EKF/1 -> SOC/1
  SOC/1 -> SOC_EKF/1  "SOC_EKF"
